simulink model "Micro_mouse"  (R2024b)
settings: Solver=FixedStepAuto  StartTime=0.0  StopTime=inf  FixedStep=0.02  RelTol=1e-3  EnableMultiTasking=on
undefined symbols (not defined in the file or in its folder): bits
libraries: stm32f4xxblockslib x10, stm32l4xxblockslib x6, simulink x5, stm32blockslib x3, slpidlib x2
settings Model: STM32="{\"PWMOutput\":[{\"ID\":\"untitled1:1\"},{\"ID\":\"Micro_mouse:1\"},{\"ID\":\"Micro_mouse:456\"},{\"ID\":\"Micro_mouse:472\"},{\"ID\":\"Micro_mouse:1057\"},{\"ID\":\"Micro_mouse:1059\"}],\"DigitalPortWrite\":[{\"ID\":\"untitled1:2\"},{\"ID\":\"Micro_mouse:2\"},{\"ID\":\"Micro_mouse:455\"},{\"ID\":\"Micro_mouse:471\"},{\"ID\":\"Micro_mouse:559\"},{\"ID\":\"Micro_mouse:1058\"},{\"ID\":\"Micro_mouse:1060\"}],\"AnalogInput\":{\"ID\":\"Micro_mouse:28\"},\"DigitalPortRead\":[{\"ID\":\"Micro_mouse:101\"},{\"ID\":\"Micro_mouse:116\"},{\"ID\":\"Micro_mouse:461\"},{\"ID\":\"Micro_mouse:462\"},{\"ID\":\"Micro_mouse:477\"},{\"ID\":\"Micro_mouse:478\"}],\"HardwareInterrupt\":[{\"ID\":\"Micro_mouse:454\"},{\"ID\":\"Micro_mouse:470\"}],\"I2CControllerRead\":{\"ID\":\"Micro_mouse:365\"},\"I2CControllerWrite\":[{\"ID\":\"Micro_mouse:366\"},{\"ID\":\"Micro_mouse:388\"}]}"  Creator=galgi  LastModifiedBy=ofekn
settings SolverCC: AutoInsertRateTranBlk=on
settings OptimizationCC: DefaultParameterBehavior=Inlined  EnhancedBackFolding=on  PassReuseOutputArgsAs=Individual arguments  ZeroExternalMemoryAtStartup=off  ZeroInternalMemoryAtStartup=off  MaxStackSize=512  OptimizeBlockOrder=speed  DifferentSizesBufferReuse=on  EfficientTunableParamExpr=on
settings DebuggingCC: ParameterTunabilityLossMsg=error
settings HardwareCC: ProdBitPerPointer=32  ProdBitPerSizeT=32  ProdBitPerPtrDiffT=32  ProdLargestAtomicInteger=Long  ProdLargestAtomicFloat=Double  ProdWordSize=32  ProdLongLongMode=on  ProdHWDeviceType=ARM Compatible->ARM Cortex-M
settings SFSimCC: MATLABDynamicMemAlloc=off
settings RTWCC: Description=Embedded Coder  SystemTargetFile=ert.tlc  HardwareBoard=STM32L4xx Based  TemplateMakefile=ert_default_tmf  Toolchain=GNU Tools for ARM Embedded Processors
settings CodeAppCC: ForceParamTrailComments=on  IgnoreCustomStorageClasses=off  OperatorAnnotations=on  SimulinkDataObjDesc=on  SFDataObjDesc=on  InsertBlockDesc=on
settings ERTTargetCC: TargetLangStandard=C99 (ISO)  CodeReplacementLibrary=ARM Cortex-M  SupportContinuousTime=on  ExtModeTransport=3  ExtModeStaticAlloc=on  ExtModeStaticAllocSize=2048  ExtModeMexFile=ext_xcp  ExtModeIntrfLevel=Level2 - Open

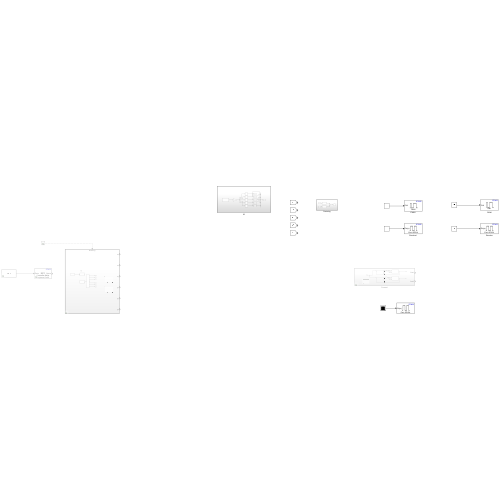
[thumbnail: Simulink's stored preview of the top-level diagram]
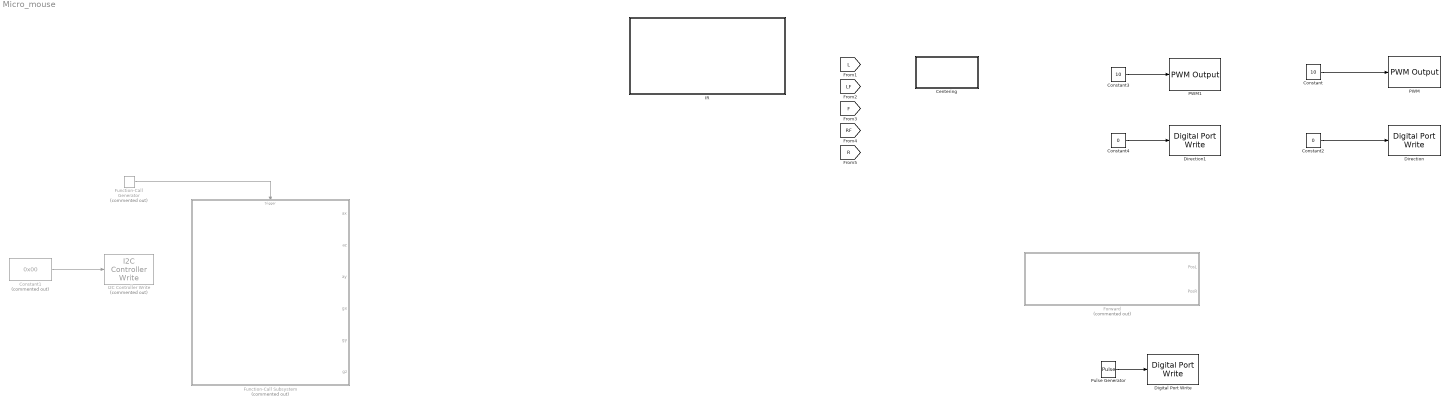
== system Micro_mouse ==
  Centering : Subsystem
  Constant : Constant  Value=10
  Constant1 : Constant  Commented=on  Value=0x00  OutDataTypeStr=uint8
  Constant2 : Constant  Value=0
  Constant3 : Constant  Value=10
  Constant4 : Constant  Value=0
  Digital Port Write : stm32f4xxblockslib/Digital Port Write  PortName=GPIOA  PinNumber=[0]  ReadOperation=off  IOAsArray=on  EnableSimPort=off  hoistedMaskSrc=ECSoC/ECSimCodegen/Digital Port Write
      settings: LibrarySourceBlock=stm32l4xxblockslib/Digital Port Write
  Direction : stm32f4xxblockslib/Digital Port Write  PortName=GPIOA  PinNumber=[11]  ReadOperation=off  IOAsArray=on  EnableSimPort=off  hoistedMaskSrc=ECSoC/ECSimCodegen/Digital Port Write
      settings: LibrarySourceBlock=stm32l4xxblockslib/Digital Port Write
  Direction1 : stm32f4xxblockslib/Digital Port Write  PortName=GPIOA  PinNumber=[12]  ReadOperation=off  IOAsArray=on  EnableSimPort=off  hoistedMaskSrc=ECSoC/ECSimCodegen/Digital Port Write
      settings: LibrarySourceBlock=stm32l4xxblockslib/Digital Port Write
  Forward : Subsystem  Commented=on
  Function-Call Generator : simulink/Ports & Subsystems/Function-Call Generator  Commented=on  sample_time=0.1  numberOfIterations=1  DisallowWideOutput=off
  Function-Call Subsystem : Subsystem  Commented=on  TreatAsAtomicUnit=on
  I2C Controller Write : stm32blockslib/I2C Controller Write  Commented=on  I2CModule=I2C1  Mode=Controller  AddressingMode=7-bits  PeripheralByteOrder=BigEndian  OwnPeripheralAddress=uint8(170)  PeripheralAddressVia=Dialog  PeripheralAddress=104  RegisterAddressMode=on  RegisterAddressVia=Dialog  RegisterAddress=107  RepeatedStart=off  NoAck=off  OutputStatus=on  BlockMode=Transmit  DataType=uint8  DataLength=1  Timeout=0.001  SampleTime=-1
      settings: LibrarySourceBlock=stm32l4xxblockslib/I2C Controller Write
  IR : Subsystem
  PWM : stm32l4xxblockslib/PWM Output  TimerModule=TIM1  DutycycleUnits=Percentage  EnableChannel1=on  EnableChannel2=off  EnableChannel3=off  EnableChannel4=off  EnableChannel5=off  EnableChannel6=off  EnableCounterInput=off  EnableMainOutputInput=off  EnableFrequencyInput=off  SetRCAfterCE=off  OutputDirection=off  OutputMainOutputEnableStatus=off  SampleTime=0.1  EnableSimPort=off  EnableUpdateEvent=off  EnableCaptureCompare1Event=off  EnableCaptureCompare2Event=off  EnableCaptureCompare3Event=off  EnableCaptureCompare4Event=off  EnableTriggerEvent=off  EnableBreakEvent=off  EnableBreakEvent2=off  ProcessorFamily=STM32L4  hoistedMaskSrc=ECSoC/ECSimCodegen/PWM Output
  PWM1 : stm32l4xxblockslib/PWM Output  TimerModule=TIM16  DutycycleUnits=Percentage  EnableChannel1=on  EnableChannel2=off  EnableChannel3=off  EnableChannel4=off  EnableChannel5=off  EnableChannel6=off  EnableCounterInput=off  EnableMainOutputInput=off  EnableFrequencyInput=off  SetRCAfterCE=off  OutputDirection=off  OutputMainOutputEnableStatus=off  SampleTime=0.1  EnableSimPort=off  EnableUpdateEvent=off  EnableCaptureCompare1Event=off  EnableCaptureCompare2Event=off  EnableCaptureCompare3Event=off  EnableCaptureCompare4Event=off  EnableTriggerEvent=off  EnableBreakEvent=off  EnableBreakEvent2=off  ProcessorFamily=STM32L4  hoistedMaskSrc=ECSoC/ECSimCodegen/PWM Output
  Pulse Generator : DiscretePulseGenerator  PulseType=Time based  PulseWidth=50
  wires:
  Function-Call Generator/1 -> Function-Call Subsystem/Trigger
  Constant1/1 -> I2C Controller Write/1
  Pulse Generator/1 -> Digital Port Write/1
  Constant/1 -> PWM/1
  Constant2/1 -> Direction/1
  Constant3/1 -> PWM1/1
  Constant4/1 -> Direction1/1

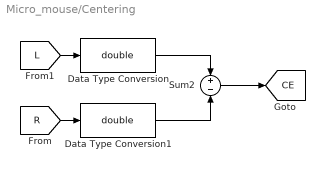
== system Micro_mouse/Centering ==
  Data Type Conversion : DataTypeConversion  OutDataTypeStr=double  SaturateOnIntegerOverflow=off  RndMeth=Floor
  Data Type Conversion1 : DataTypeConversion  OutDataTypeStr=double  SaturateOnIntegerOverflow=off  RndMeth=Floor
  Sum2 : Sum  Inputs=+|-
  tag scope: CE=global
  wires:
  [R] -> Data Type Conversion1/1
  [L] -> Data Type Conversion/1
  Sum2/1 -> [CE]
  Data Type Conversion/1 -> Sum2/1
  Data Type Conversion1/1 -> Sum2/2

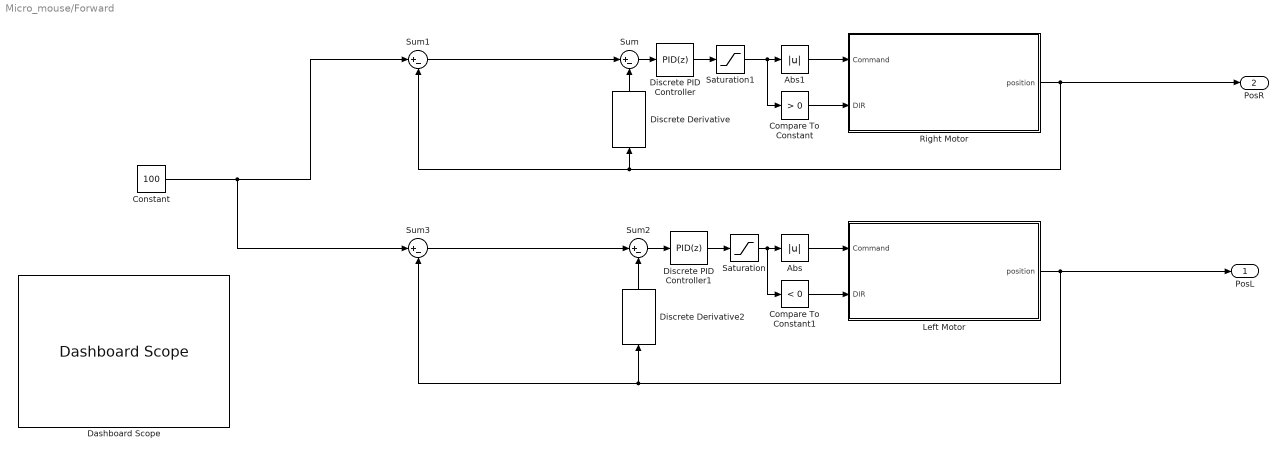
== system Micro_mouse/Forward ==
  Abs : Abs  SaturateOnIntegerOverflow=off
  Abs1 : Abs  SaturateOnIntegerOverflow=off
  Compare To Constant : simulink/Logic and Bit Operations/Compare To Constant  relop=>  const=0  OutDataTypeStr=boolean
  Compare To Constant1 : simulink/Logic and Bit Operations/Compare To Constant  relop=<  const=0  OutDataTypeStr=boolean
  Constant : Constant  Value=100
  Dashboard Scope : DashboardScope
  Discrete Derivative : simulink/Discrete/Discrete Derivative  gainval=1.0  ICPrevScaledInput=0.0  OutMin=[]  OutMax=[]  OutDataType=fixdt(1, 16)  OutScaling=2^-10  DoSatur=off
  Discrete Derivative2 : simulink/Discrete/Discrete Derivative  gainval=1.0  ICPrevScaledInput=0.0  OutMin=[]  OutMax=[]  OutDataType=fixdt(1, 16)  OutScaling=2^-10  DoSatur=off
  Discrete PID Controller : slpidlib/PID Controller  Controller=PID  Form=Parallel  TimeDomain=Discrete-time  UseExternalTs=off  SampleTime=-1  IntegratorMethod=Forward Euler  FilterMethod=Forward Euler  ControllerParametersSource=internal  P=5  I=1  UseKiTs=off  D=0  UseExternalDerivativeSource=off  N=100  UseFilter=on  TunerSelectOption=Transfer Function Based (PID Tuner App)  InitialConditionSource=internal  InitialConditionForIntegrator=0  InitialConditionForFilter=0  DifferentiatorICPrevScaledInput=0  ExternalReset=none  TrackingMode=off  Kt=1  LimitOutput=off  SatLimitsSource=internal  UpperSaturationLimit=inf  LowerSaturationLimit=-inf  LinearizeAsGain=off  AntiWindupMode=none  Kb=1  LimitIntegrator=off  UpperIntegratorSaturationLimit=inf  LowerIntegratorSaturationLimit=-inf  POutMin=[]  POutMax=[]  IOutMin=[]  IOutMax=[]  DOutMin=[]  DOutMax=[]  NOutMin=[]  NOutMax=[]  SumOutMin=[]  SumOutMax=[]  SaturationOutMin=[]  SaturationOutMax=[]  PParamMin=[]  PParamMax=[]  IParamMin=[]  IParamMax=[]  DParamMin=[]  DParamMax=[]  NParamMin=[]  NParamMax=[]  KbParamMin=[]  KbParamMax=[]  KtParamMin=[]  KtParamMax=[]  KbOutMin=[]  KbOutMax=[]  KtOutMin=[]  KtOutMax=[]  IntegratorOutMin=[]  IntegratorOutMax=[]  FilterOutMin=[]  FilterOutMax=[]  SumI1OutMin=[]  SumI1OutMax=[]  SumI2OutMin=[]  SumI2OutMax=[]  SumI3OutMin=[]  SumI3OutMax=[]  SumI4OutMin=[]  SumI4OutMax=[]  SumDOutMin=[]  SumDOutMax=[]  DifferentiatorOutMin=[]  DifferentiatorOutMax=[]  FilterDiffOutCoefMin=[]  FilterDiffOutCoefMax=[]  ReciprocalOutMin=[]  ReciprocalOutMax=[]  SumDenOutMin=[]  SumDenOutMax=[]  SumNumOutMin=[]  SumNumOutMax=[]  DivideOutMin=[]  DivideOutMax=[]  UdiffTsProdOutMin=[]  UdiffTsProdOutMax=[]  NTsProdOutMin=[]  NTsProdOutMax=[]  UintegralTsProdOutMin=[]  UintegralTsProdOutMax=[]  UngainTsProdOutMin=[]  UngainTsProdOutMax=[]  ClampingZeroOutDataTypeStr=Inherit: Inherit via back propagation  ClampingZeroOutMin=[]  ClampingZeroOutMax=[]  FilterDenConstantOutDataTypeStr=Inherit: Inherit via back propagation  FilterDenConstantOutMin=[]  FilterDenConstantOutMax=[]  PCopyOutDataTypeStr=Inherit: Inherit via back propagation  PCopyOutMin=[]  PCopyOutMax=[]  NCopyOutDataTypeStr=Inherit: Inherit via back propagation  NCopyOutMin=[]  NCopyOutMax=[]  IntegratorContinuousStateAttributes=''  IntegratorStateMustResolveToSignalObject=off  IntegratorRTWStateStorageClass=Auto  FilterContinuousStateAttributes=''  FilterStateMustResolveToSignalObject=off  FilterRTWStateStorageClass=Auto  ParallelPVariant=InternalParameters  IdealPVariant=Disabled  IVariant=InternalParameters  DVariant=InternalParameters  IntegratorVariant=Discrete  SatVariant=Disabled  AWVariant=Passthrough  PCopyVariant=Disabled  TRVariant=Disabled  FdbkBlocksVariant=Forward  IdealPFdbkVariant=Disabled  SatFdbkVariant=Disabled  DerivativeFilterVariant=ForwardEulerFilter  NVariant=InternalParameters  NCopyVariant=Disabled  FilterICVariant=InternalICsFilter  IntegratorICVariant=InternalICs  ExternalResetVariant=Disabled  TRSumVariant=Passthrough  SumFdbkVariant=Disabled  SumVariant=Sum_PID  TsampFilterVariant=InternalTs  TsampNgainVariant=Passthrough  TsampIntegralVariant=Disabled_SignalSpec  ExternalSaturationOutDataTypeStr=Inherit: Same as second input  DerivativeSourceVariant=ErrorSignal  PreIntVariant=InternalPreInt
      settings: LibrarySourceBlock=simulink/Discrete/Discrete PID Controller
  Discrete PID Controller1 : slpidlib/PID Controller  Controller=PID  Form=Parallel  TimeDomain=Discrete-time  UseExternalTs=off  SampleTime=-1  IntegratorMethod=Forward Euler  FilterMethod=Forward Euler  ControllerParametersSource=internal  P=5  I=1  UseKiTs=off  D=0  UseExternalDerivativeSource=off  N=100  UseFilter=on  TunerSelectOption=Transfer Function Based (PID Tuner App)  InitialConditionSource=internal  InitialConditionForIntegrator=0  InitialConditionForFilter=0  DifferentiatorICPrevScaledInput=0  ExternalReset=none  TrackingMode=off  Kt=1  LimitOutput=off  SatLimitsSource=internal  UpperSaturationLimit=inf  LowerSaturationLimit=-inf  LinearizeAsGain=off  AntiWindupMode=none  Kb=1  LimitIntegrator=off  UpperIntegratorSaturationLimit=inf  LowerIntegratorSaturationLimit=-inf  POutMin=[]  POutMax=[]  IOutMin=[]  IOutMax=[]  DOutMin=[]  DOutMax=[]  NOutMin=[]  NOutMax=[]  SumOutMin=[]  SumOutMax=[]  SaturationOutMin=[]  SaturationOutMax=[]  PParamMin=[]  PParamMax=[]  IParamMin=[]  IParamMax=[]  DParamMin=[]  DParamMax=[]  NParamMin=[]  NParamMax=[]  KbParamMin=[]  KbParamMax=[]  KtParamMin=[]  KtParamMax=[]  KbOutMin=[]  KbOutMax=[]  KtOutMin=[]  KtOutMax=[]  IntegratorOutMin=[]  IntegratorOutMax=[]  FilterOutMin=[]  FilterOutMax=[]  SumI1OutMin=[]  SumI1OutMax=[]  SumI2OutMin=[]  SumI2OutMax=[]  SumI3OutMin=[]  SumI3OutMax=[]  SumI4OutMin=[]  SumI4OutMax=[]  SumDOutMin=[]  SumDOutMax=[]  DifferentiatorOutMin=[]  DifferentiatorOutMax=[]  FilterDiffOutCoefMin=[]  FilterDiffOutCoefMax=[]  ReciprocalOutMin=[]  ReciprocalOutMax=[]  SumDenOutMin=[]  SumDenOutMax=[]  SumNumOutMin=[]  SumNumOutMax=[]  DivideOutMin=[]  DivideOutMax=[]  UdiffTsProdOutMin=[]  UdiffTsProdOutMax=[]  NTsProdOutMin=[]  NTsProdOutMax=[]  UintegralTsProdOutMin=[]  UintegralTsProdOutMax=[]  UngainTsProdOutMin=[]  UngainTsProdOutMax=[]  ClampingZeroOutDataTypeStr=Inherit: Inherit via back propagation  ClampingZeroOutMin=[]  ClampingZeroOutMax=[]  FilterDenConstantOutDataTypeStr=Inherit: Inherit via back propagation  FilterDenConstantOutMin=[]  FilterDenConstantOutMax=[]  PCopyOutDataTypeStr=Inherit: Inherit via back propagation  PCopyOutMin=[]  PCopyOutMax=[]  NCopyOutDataTypeStr=Inherit: Inherit via back propagation  NCopyOutMin=[]  NCopyOutMax=[]  IntegratorContinuousStateAttributes=''  IntegratorStateMustResolveToSignalObject=off  IntegratorRTWStateStorageClass=Auto  FilterContinuousStateAttributes=''  FilterStateMustResolveToSignalObject=off  FilterRTWStateStorageClass=Auto  ParallelPVariant=InternalParameters  IdealPVariant=Disabled  IVariant=InternalParameters  DVariant=InternalParameters  IntegratorVariant=Discrete  SatVariant=Disabled  AWVariant=Passthrough  PCopyVariant=Disabled  TRVariant=Disabled  FdbkBlocksVariant=Forward  IdealPFdbkVariant=Disabled  SatFdbkVariant=Disabled  DerivativeFilterVariant=ForwardEulerFilter  NVariant=InternalParameters  NCopyVariant=Disabled  FilterICVariant=InternalICsFilter  IntegratorICVariant=InternalICs  ExternalResetVariant=Disabled  TRSumVariant=Passthrough  SumFdbkVariant=Disabled  SumVariant=Sum_PID  TsampFilterVariant=InternalTs  TsampNgainVariant=Passthrough  TsampIntegralVariant=Disabled_SignalSpec  ExternalSaturationOutDataTypeStr=Inherit: Same as second input  DerivativeSourceVariant=ErrorSignal  PreIntVariant=InternalPreInt
      settings: LibrarySourceBlock=simulink/Discrete/Discrete PID Controller
  Left Motor : Subsystem
  Right Motor : Subsystem
  Saturation : Saturate  UpperLimit=100  LowerLimit=-100
  Saturation1 : Saturate  UpperLimit=99  LowerLimit=-99
  Sum{,1..3} (4 alike) : Sum  Inputs=|+-
  PosL : Outport
  PosR : Outport  Port=2
  wires:
  Discrete Derivative/1 -> Sum/2
  Right Motor/1(position) -> PosR/1, Discrete Derivative/1, Sum1/2
  Left Motor/1(position) -> PosL/1, Discrete Derivative2/1, Sum3/2
  Saturation1/1 -> Compare To Constant/1, Abs1/1
  Discrete Derivative2/1 -> Sum2/2
  Compare To Constant/1 -> Right Motor/2(DIR)
  Saturation/1 -> Compare To Constant1/1, Abs/1
  Abs/1 -> Left Motor/1(Command)
  Abs1/1 -> Right Motor/1(Command)
  Compare To Constant1/1 -> Left Motor/2(DIR)
  Sum1/1 -> Sum/1
  Sum3/1 -> Sum2/1
  Sum/1 -> Discrete PID Controller/1
  Discrete PID Controller/1 -> Saturation1/1
  Discrete PID Controller1/1 -> Saturation/1
  Sum2/1 -> Discrete PID Controller1/1
  Constant/1 -> Sum3/1, Sum1/1

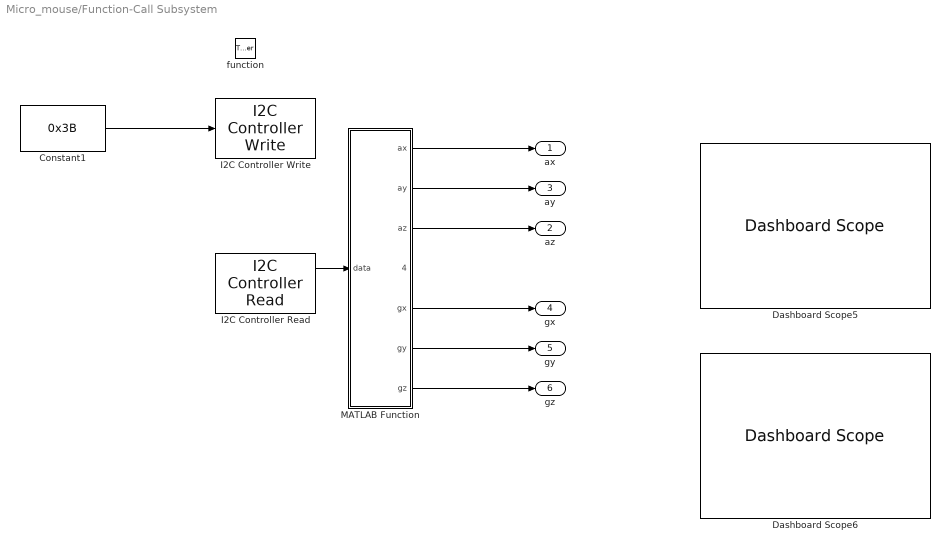
== system Micro_mouse/Function-Call Subsystem ==
  function : TriggerPort  TriggerType=function-call  VariantControl=(inherit)
  Constant1 : Constant  Value=0x3B  OutDataTypeStr=uint8
  Dashboard Scope5 : DashboardScope
  Dashboard Scope6 : DashboardScope
  I2C Controller Read : stm32blockslib/I2C Controller Read  I2CModule=I2C1  Mode=Controller  AddressingMode=7-bits  PeripheralByteOrder=BigEndian  OwnPeripheralAddress=uint8(170)  PeripheralAddressVia=Dialog  PeripheralAddress=104  RegisterAddressMode=on  RegisterAddressVia=Dialog  RegisterAddress=59  RepeatedStart=off  NoAck=off  OutputStatus=on  BlockMode=Receive  DataType=uint8  DataLength=14  Timeout=0.001  SampleTime=-1
      settings: LibrarySourceBlock=stm32l4xxblockslib/I2C Controller Read
  I2C Controller Write : stm32blockslib/I2C Controller Write  I2CModule=I2C1  Mode=Controller  AddressingMode=7-bits  PeripheralByteOrder=BigEndian  OwnPeripheralAddress=uint8(170)  PeripheralAddressVia=Dialog  PeripheralAddress=104  RegisterAddressMode=on  RegisterAddressVia=Dialog  RegisterAddress=107  RepeatedStart=off  NoAck=off  OutputStatus=on  BlockMode=Transmit  DataType=uint8  DataLength=1  Timeout=0.001  SampleTime=-1
      settings: LibrarySourceBlock=stm32l4xxblockslib/I2C Controller Write
  MATLAB Function : MATLAB Function  TreatAsAtomicUnit=on
  ax : Outport
  az : Outport  Port=2
  ay : Outport  Port=3
  gx : Outport  Port=4
  gy : Outport  Port=5
  gz : Outport  Port=6
  wires:
  MATLAB Function/2(ay) -> ay/1
  MATLAB Function/6(gy) -> gy/1
  Constant1/1 -> I2C Controller Write/1
  MATLAB Function/7(gz) -> gz/1
  MATLAB Function/1(ax) -> ax/1
  MATLAB Function/3(az) -> az/1
  I2C Controller Read/1 -> MATLAB Function/1(data)
  MATLAB Function/5(gx) -> gx/1

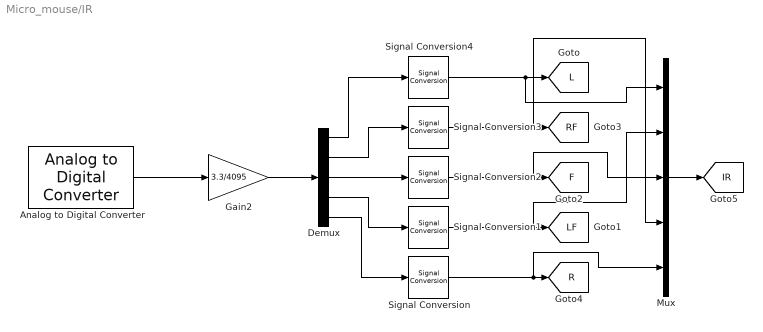
== system Micro_mouse/IR ==
  Analog to Digital Converter : stm32f4xxblockslib/Analog to Digital Converter  ADCModule=ADC1  ConversionGroup=Regular  TriggerMode=Trigger and read  NumberOfConversions=5  EnableBufferConv=off  BufferLength=1  OutputStatus=off  SampleTime=-1  EnableSimPort=off  hoistedMaskSrc=ECSoC/ECSimCodegen/Analog to Digital Converter
      settings: LibrarySourceBlock=stm32l4xxblockslib/Analog to Digital Converter
  Demux : Demux  Outputs=5
  Gain2 : Gain  Gain=3.3/4095
  Mux : Mux  Inputs=5
  Signal Conversion{,1..4} (5 alike) : SignalConversion  OverrideOpt=off
  tag scope: F=global, IR=global, L=global, LF=global, R=global, RF=global
  wires:
  Demux/3 -> Signal Conversion2/1
  Demux/5 -> Signal Conversion/1
  Demux/4 -> Signal Conversion1/1
  Signal Conversion3/1 -> Mux/4, [RF]
  Analog to Digital Converter/1 -> Gain2/1
  Gain2/1 -> Demux/1
  Demux/2 -> Signal Conversion3/1
  Demux/1 -> Signal Conversion4/1
  Signal Conversion2/1 -> Mux/3, [F]
  Signal Conversion/1 -> Mux/5, [R]
  Signal Conversion1/1 -> Mux/2, [LF]
  Signal Conversion4/1 -> Mux/1, [L]
  Mux/1 -> [IR]

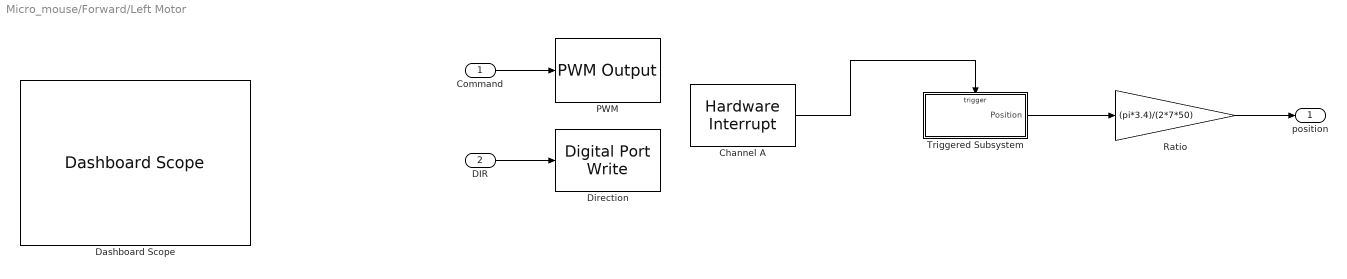
== system Micro_mouse/Forward/Left Motor ==
  Command : Inport
  DIR : Inport  Port=2
  Channel A : stm32l4xxblockslib/Hardware Interrupt  ISRGroup=External interrupts (EXTI)  ISRName=EXTI3_IRQHandler  ISRNumber=24  EventsList={ 'on', 'EXTI3 Event', '1'; 'off', 'Custom event', '2' }  SelectedEvents={'EXTI3 Event'}  TaskPriority=30  DisablePreemption=off  ClearInterruptFlagsAtEndOfEvent=off  InterruptDefinitionFile=$(TARGET_ROOT)/registry/interrupts/STM32F4xxBased_interrupts.xml  HardwareBoard=STM32L4xx Based  EnableSimPort=off
  Dashboard Scope : DashboardScope
  Direction : stm32f4xxblockslib/Digital Port Write  PortName=GPIOA  PinNumber=[12]  ReadOperation=off  IOAsArray=on  EnableSimPort=off  hoistedMaskSrc=ECSoC/ECSimCodegen/Digital Port Write
      settings: LibrarySourceBlock=stm32l4xxblockslib/Digital Port Write
  PWM : stm32l4xxblockslib/PWM Output  TimerModule=TIM16  DutycycleUnits=Percentage  EnableChannel1=on  EnableChannel2=off  EnableChannel3=off  EnableChannel4=off  EnableChannel5=off  EnableChannel6=off  EnableCounterInput=off  EnableMainOutputInput=off  EnableFrequencyInput=off  SetRCAfterCE=off  OutputDirection=off  OutputMainOutputEnableStatus=off  SampleTime=0.1  EnableSimPort=off  EnableUpdateEvent=off  EnableCaptureCompare1Event=off  EnableCaptureCompare2Event=off  EnableCaptureCompare3Event=off  EnableCaptureCompare4Event=off  EnableTriggerEvent=off  EnableBreakEvent=off  EnableBreakEvent2=off  ProcessorFamily=STM32L4  hoistedMaskSrc=ECSoC/ECSimCodegen/PWM Output
  Ratio : Gain  Gain=(pi*3.4)/(2*7*50)
  Triggered Subsystem : Subsystem  TreatAsAtomicUnit=on
  position : Outport
  wires:
  Command/1 -> PWM/1
  Triggered Subsystem/1(Position) -> Ratio/1
  Channel A/1 -> Triggered Subsystem/Trigger
  Ratio/1 -> position/1
  DIR/1 -> Direction/1

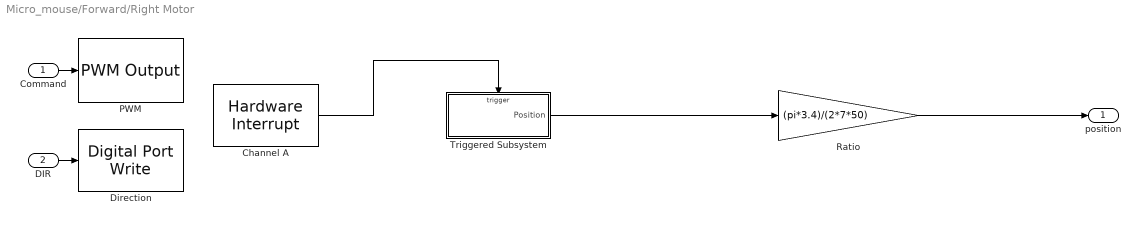
== system Micro_mouse/Forward/Right Motor ==
  Command : Inport
  DIR : Inport  Port=2
  Channel A : stm32l4xxblockslib/Hardware Interrupt  ISRGroup=External interrupts (EXTI)  ISRName=EXTI0_IRQHandler  ISRNumber=21  EventsList={ 'on', 'EXTI0 Event', '1'; 'off', 'Custom event', '2' }  SelectedEvents={'EXTI0 Event'}  TaskPriority=30  DisablePreemption=off  ClearInterruptFlagsAtEndOfEvent=off  InterruptDefinitionFile=$(TARGET_ROOT)/registry/interrupts/STM32F4xxBased_interrupts.xml  HardwareBoard=STM32L4xx Based  EnableSimPort=off
  Direction : stm32f4xxblockslib/Digital Port Write  PortName=GPIOA  PinNumber=[11]  ReadOperation=off  IOAsArray=on  EnableSimPort=off  hoistedMaskSrc=ECSoC/ECSimCodegen/Digital Port Write
      settings: LibrarySourceBlock=stm32l4xxblockslib/Digital Port Write
  PWM : stm32l4xxblockslib/PWM Output  TimerModule=TIM1  DutycycleUnits=Percentage  EnableChannel1=on  EnableChannel2=off  EnableChannel3=off  EnableChannel4=off  EnableChannel5=off  EnableChannel6=off  EnableCounterInput=off  EnableMainOutputInput=off  EnableFrequencyInput=off  SetRCAfterCE=off  OutputDirection=off  OutputMainOutputEnableStatus=off  SampleTime=0.1  EnableSimPort=off  EnableUpdateEvent=off  EnableCaptureCompare1Event=off  EnableCaptureCompare2Event=off  EnableCaptureCompare3Event=off  EnableCaptureCompare4Event=off  EnableTriggerEvent=off  EnableBreakEvent=off  EnableBreakEvent2=off  ProcessorFamily=STM32L4  hoistedMaskSrc=ECSoC/ECSimCodegen/PWM Output
  Ratio : Gain  Gain=(pi*3.4)/(2*7*50)
  Triggered Subsystem : Subsystem  TreatAsAtomicUnit=on
  position : Outport
  wires:
  Command/1 -> PWM/1
  DIR/1 -> Direction/1
  Channel A/1 -> Triggered Subsystem/Trigger
  Ratio/1 -> position/1
  Triggered Subsystem/1(Position) -> Ratio/1

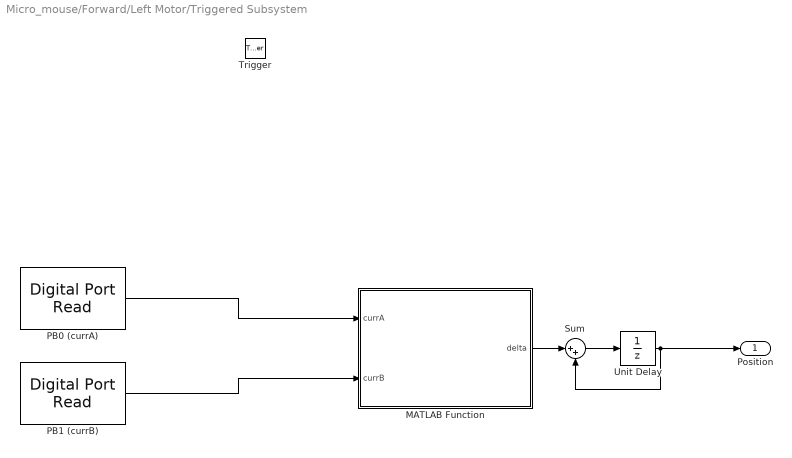
== system Micro_mouse/Forward/Left Motor/Triggered Subsystem ==
  Trigger : TriggerPort  TriggerType=function-call  VariantControl=(inherit)
  MATLAB Function : MATLAB Function  TreatAsAtomicUnit=on
  PB0 (currA) : stm32f4xxblockslib/Digital Port Read  PortName=GPIOB  PinNumber=[3]  ReadOperation=on  IOAsArray=on  SampleTime=-1  EnableSimPort=off  hoistedMaskSrc=ECSoC/ECSimCodegen/Digital Port Read
      settings: LibrarySourceBlock=stm32l4xxblockslib/Digital Port Read
  PB1 (currB) : stm32f4xxblockslib/Digital Port Read  PortName=GPIOB  PinNumber=[4]  ReadOperation=on  IOAsArray=on  SampleTime=-1  EnableSimPort=off  hoistedMaskSrc=ECSoC/ECSimCodegen/Digital Port Read
      settings: LibrarySourceBlock=stm32l4xxblockslib/Digital Port Read
  Sum : Sum  Inputs=|++
  Unit Delay : UnitDelay  SampleTime=-1  HasFrameUpgradeWarning=on
  Position : Outport
  wires:
  PB1 (currB)/1 -> MATLAB Function/2(currB)
  PB0 (currA)/1 -> MATLAB Function/1(currA)
  Unit Delay/1 -> Sum/2, Position/1
  Sum/1 -> Unit Delay/1
  MATLAB Function/1(delta) -> Sum/1

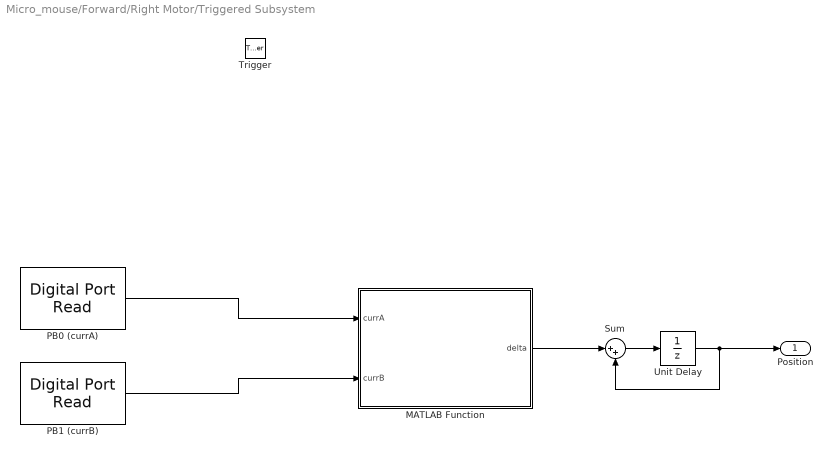
== system Micro_mouse/Forward/Right Motor/Triggered Subsystem ==
  Trigger : TriggerPort  TriggerType=function-call  VariantControl=(inherit)
  MATLAB Function : MATLAB Function  TreatAsAtomicUnit=on
  PB0 (currA) : stm32f4xxblockslib/Digital Port Read  PortName=GPIOB  PinNumber=[0]  ReadOperation=on  IOAsArray=on  SampleTime=-1  EnableSimPort=off  hoistedMaskSrc=ECSoC/ECSimCodegen/Digital Port Read
      settings: LibrarySourceBlock=stm32l4xxblockslib/Digital Port Read
  PB1 (currB) : stm32f4xxblockslib/Digital Port Read  PortName=GPIOB  PinNumber=[1]  ReadOperation=on  IOAsArray=on  SampleTime=-1  EnableSimPort=off  hoistedMaskSrc=ECSoC/ECSimCodegen/Digital Port Read
      settings: LibrarySourceBlock=stm32l4xxblockslib/Digital Port Read
  Sum : Sum  Inputs=|++
  Unit Delay : UnitDelay  SampleTime=-1  HasFrameUpgradeWarning=on
  Position : Outport
  wires:
  PB1 (currB)/1 -> MATLAB Function/2(currB)
  PB0 (currA)/1 -> MATLAB Function/1(currA)
  Unit Delay/1 -> Sum/2, Position/1
  Sum/1 -> Unit Delay/1
  MATLAB Function/1(delta) -> Sum/1

== matlab function Micro_mouse/Function-Call Subsystem/MATLAB Function ==
  data: data input; ax output int16 size=1; ay output int16 size=1; az output int16 size=1; tempC output double size=1; gx output int16 size=1; gy output int16 size=1; gz output int16 size=1
function [ax, ay, az, tempC, gx, gy, gz] = decodeMPU(data)
%#codegen
% data must be [14x1] uint8 externally defined

ax = typecast([data(1), data(2)], 'int16');
ay = typecast([data(3), data(4)], 'int16');
az = typecast([data(5), data(6)], 'int16');

t = typecast([data(7), data(8)], 'int16');
tempC = double(t) / 333.87 + 21.0;

gx = typecast([data(9),  data(10)], 'int16');
gy = typecast([data(11), data(12)], 'int16');
gz = typecast([data(13), data(14)], 'int16');
end

== matlab function Micro_mouse/Forward/Left Motor/Triggered Subsystem/MATLAB Function ==
  data: delta output; currA input; currB input
function delta = decodeSimple(currA, currB)
    if (currA == currB)
        delta = +1;   % Forward
    else
        delta = -1;   % Reverse
    end
end

== matlab function Micro_mouse/Forward/Right Motor/Triggered Subsystem/MATLAB Function ==
  data: delta output; currA input; currB input
function delta = decodeSimple(currA, currB)
    if (currA == currB)
        delta = -1;   % Forward
    else
        delta = +1;   % Reverse
    end
end
